simulink model "Modello_non_lineare_Hinfsyn"  (R2022b)
settings: Solver=VariableStepAuto  StartTime=0.0  StopTime=60  RelTol=1e-3
values from neighbouring files (symbols this model uses):
  Km = 1.08    [Inizializzazione_segway.m]
  Tm = 0.005    [Inizializzazione_segway.m]
undefined symbols (not defined in the file or in its folder): K_ms, K_musyn
libraries: simulink x2
settings Model: Creator=anton  LastModifiedBy=angel

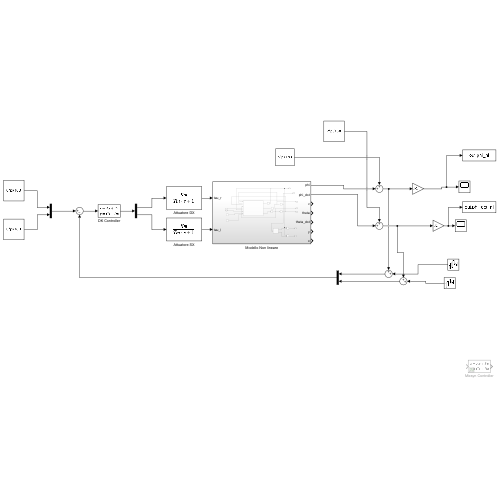
[thumbnail: Simulink's stored preview of the top-level diagram]
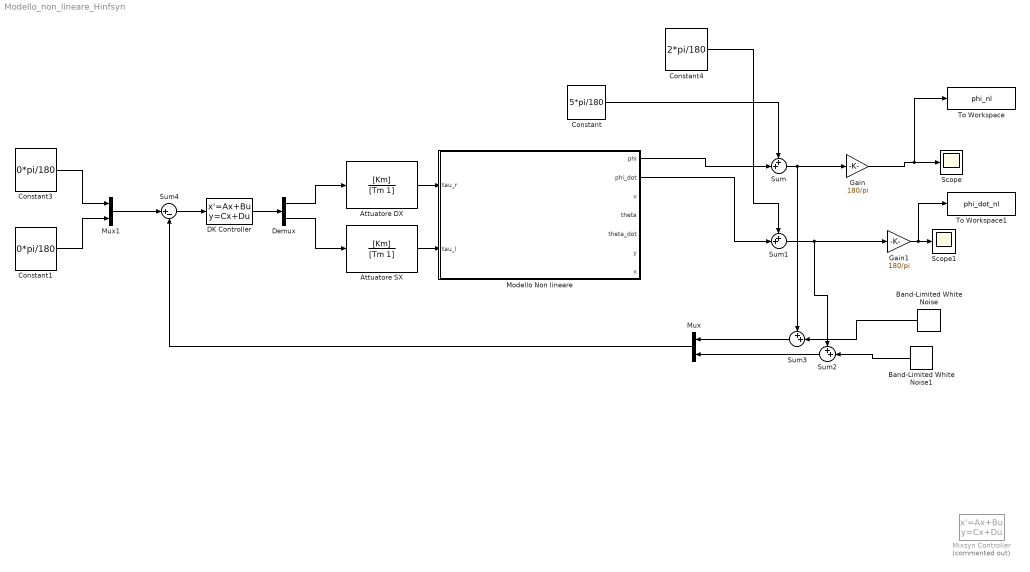
== system Modello_non_lineare_Hinfsyn ==
  Attuatore DX : TransferFcn  Numerator=[Km]  Denominator=[Tm 1]
  Attuatore SX : TransferFcn  Numerator=[Km]  Denominator=[Tm 1]
  Band-Limited White Noise : simulink/Sources/Band-Limited White Noise  Cov=[0.001]  Ts=0.1  seed=[23341]
  Band-Limited White Noise1 : simulink/Sources/Band-Limited White Noise  Cov=[0.001]  Ts=0.1  seed=[23341]
  Constant : Constant  Value=5*pi/180
  Constant1 : Constant  Value=0*pi/180
  Constant3 : Constant  Value=0*pi/180
  Constant4 : Constant  Value=2*pi/180
  DK Controller : StateSpace  A=K_musyn.A  B=K_musyn.B  C=K_musyn.C  D=K_musyn.D  InitialCondition=zeros(length(K_musyn.A),1)
  Demux : Demux  Outputs=2
  Gain : Gain  Gain=180/pi
  Gain1 : Gain  Gain=180/pi
  Mixsyn Controller : StateSpace  Commented=on  A=K_ms.A  B=K_ms.B  C=K_ms.C  D=K_ms.D  InitialCondition=zeros(length(K_ms.A),1)
  Modello Non lineare : Subsystem
  Mux : Mux  Inputs=2
  Mux1 : Mux  Inputs=2
  Scope : Scope
  Scope1 : Scope
  Sum{,1..3} (4 alike) : Sum  Inputs=++|
  Sum4 : Sum  Inputs=|+-
  To Workspace : ToWorkspace  VariableName=phi_nl  SaveFormat=Timeseries  SampleTime=-1
  To Workspace1 : ToWorkspace  VariableName=phi_dot_nl  SaveFormat=Timeseries  SampleTime=-1
  wires:
  Modello Non lineare/2(phi_dot) -> Sum1/2
  Attuatore SX/1 -> Modello Non lineare/2(tau_l)
  Attuatore DX/1 -> Modello Non lineare/1(tau_r)
  Demux/1 -> Attuatore DX/1
  Demux/2 -> Attuatore SX/1
  Sum/1 -> Gain/1, Sum3/1
  Sum1/1 -> Sum2/1, Gain1/1
  Modello Non lineare/1(phi) -> Sum/2
  Mux/1 -> Sum4/2
  Constant3/1 -> Mux1/1
  Constant1/1 -> Mux1/2
  Mux1/1 -> Sum4/1
  Sum3/1 -> Mux/1
  Sum2/1 -> Mux/2
  Gain/1 -> To Workspace/1, Scope/1
  Gain1/1 -> To Workspace1/1, Scope1/1
  Constant4/1 -> Sum1/1
  Constant/1 -> Sum/1
  Sum4/1 -> DK Controller/1
  DK Controller/1 -> Demux/1
  Band-Limited White Noise/1 -> Sum3/2
  Band-Limited White Noise1/1 -> Sum2/2

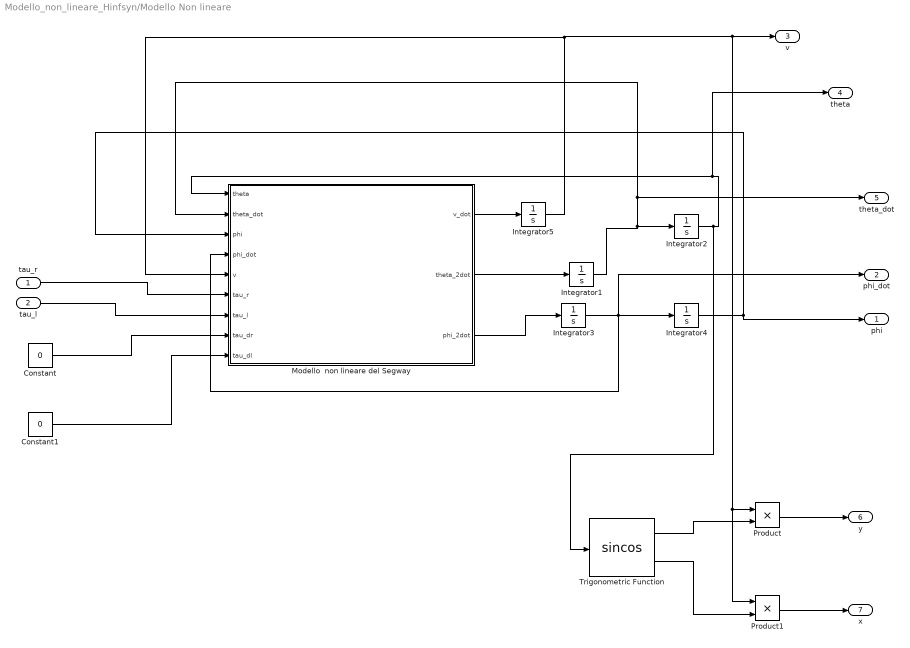
== system Modello_non_lineare_Hinfsyn/Modello Non lineare ==
  tau_r : Inport
  tau_l : Inport  Port=2
  Constant : Constant  Value=0
  Constant1 : Constant  Value=0
  Integrator{1..5} (5 alike) : Integrator
  Modello  non lineare del Segway : MATLAB Function  TreatAsAtomicUnit=on
  Product : Product
  Product1 : Product
  Trigonometric Function : Trigonometry  Operator=sincos
  phi : Outport
  phi_dot : Outport  Port=2
  v : Outport  Port=3
  theta : Outport  Port=4
  theta_dot : Outport  Port=5
  y : Outport  Port=6
  x : Outport  Port=7
  wires:
  Modello  non lineare del Segway/2(theta_2dot) -> Integrator1/1
  Modello  non lineare del Segway/3(phi_2dot) -> Integrator3/1
  Integrator4/1 -> phi/1, Modello  non lineare del Segway/3(phi)
  tau_l/1 -> Modello  non lineare del Segway/7(tau_l)
  Integrator3/1 -> phi_dot/1, Modello  non lineare del Segway/4(phi_dot), Integrator4/1
  tau_r/1 -> Modello  non lineare del Segway/6(tau_r)
  Integrator2/1 -> Trigonometric Function/1, theta/1, Modello  non lineare del Segway/1(theta)
  Integrator1/1 -> Integrator2/1, theta_dot/1, Modello  non lineare del Segway/2(theta_dot)
  Modello  non lineare del Segway/1(v_dot) -> Integrator5/1
  Integrator5/1 -> Product1/1, Product/1, v/1, Modello  non lineare del Segway/5(v)
  Trigonometric Function/1 -> Product/2
  Trigonometric Function/2 -> Product1/2
  Product/1 -> y/1
  Product1/1 -> x/1
  Constant/1 -> Modello  non lineare del Segway/8(tau_dr)
  Constant1/1 -> Modello  non lineare del Segway/9(tau_dl)

== matlab function Modello_non_lineare_Hinfsyn/Modello Non lineare/Modello  non lineare del Segway ==
  data: v_dot output; theta input; theta_dot input; phi input; phi_dot input; v input; tau_r input; tau_l input; theta_2dot output; phi_2dot output; tau_dr input; tau_dl input
function [v_dot, theta_2dot, phi_2dot] = SegwayDynamics(theta, theta_dot, phi, ...
    phi_dot, v, tau_r, tau_l, tau_dr, tau_dl)
    
    g = 9.81;
    m = 1.22;
    r = 0.13;
    a = 0.496/2;
    L = 0.2924;
    g = 9.81;
    M = 54;

    M_vdot = 2*(3/2*m +0.5*M);
    M_theta2dot = 2*(3/2*m*a^2 + 1/6*M*a^2 + 1/2*M*L^2*sin(phi)^2);
    M_phi2dot = 2*(1/2*m*r^2 + 2/3*M*L^2);
    M_vdot_phi2dot = -m*r+M*L*cos(phi);
    c_v = -M*L*sin(phi)*(theta_dot^2 + phi_dot^2);
    c_thetadot = 2*M*L^2*sin(phi)*cos(phi)*theta_dot*phi_dot+M*L*sin(phi)...
                    *v*theta_dot;
    c_phidot = -M*L^2*sin(phi)*cos(phi)*theta_dot^2;
    g_phidot = -M*L*g*sin(phi);
    
    I = [M_vdot 0 M_vdot_phi2dot;
         0 M_theta2dot 0;
         M_vdot_phi2dot 0 M_phi2dot];
    
    C = [c_v c_thetadot c_phidot]';
    G = [0 0 g_phidot]';
    
    Ing = [1/r 1/r;
           a/r -a/r;
           -1 -1];

    csi567_dot = inv(I)*(Ing*[tau_r + tau_dr,tau_l + tau_dl]' - C -G);
    v_dot = csi567_dot(1);
    theta_2dot = csi567_dot(2);
    phi_2dot = csi567_dot(3);
